simulink model "sim_noise_reduction_R2013a"  (R2013a)
settings: Solver=ode4  SolverMode=SingleTasking  StartTime=0.0  StopTime=10.0  FixedStep=0.001  RelTol=1e-3
libraries: simulink x1
settings Model: CovMetricSettings=dwe  CovHtmlReporting=off  covSaveCumulativeToWorkspaceVar=off  CovSaveSingleToWorkspaceVar=off  CovExternalEMLEnable=on  Creator=kawata  LastModifiedBy=kawata
settings DataIOCC: LimitDataPoints=off  SaveFormat=StructureWithTime
settings DebuggingCC: UnderspecifiedInitializationDetection=Simplified  MergeDetectMultiDrivingBlocksExec=error  SolverPrmCheckMsg=none  FrameProcessingCompatibilityMsg=error  StateNameClashWarn=none  SFUnexpectedBacktrackingDiag=error  SFNoUnconditionalDefaultTransitionDiag=error
settings HardwareCC: ProdBitPerPointer=64  ProdLargestAtomicFloat=Float  ProdIntDivRoundTo=Zero  ProdEndianess=LittleEndian  ProdHWDeviceType=Specified
settings ModelReferenceCC: PropagateSignalLabelsOutOfModel=on
settings GRTTargetCC: CodeReplacementLibrary=C99 (ISO)  GeneratePreprocessorConditionals=Use local settings

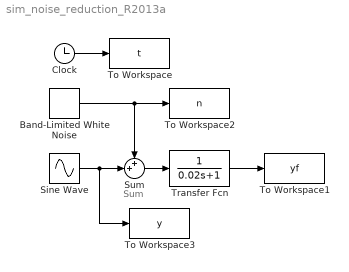
== system sim_noise_reduction_R2013a ==
  note: Sum
  Band-Limited White Noise : simulink/Sources/Band-Limited White Noise  Cov=[1e-5]  Ts=0.001  seed=[23341]
  Clock : Clock
  Sine Wave : Sin  SampleTime=0
  Sum : Sum  Inputs=++|
  To Workspace : ToWorkspace  VariableName=t  SampleTime=-1
  To Workspace1 : ToWorkspace  VariableName=yf  SampleTime=-1
  To Workspace2 : ToWorkspace  VariableName=n  SampleTime=-1
  To Workspace3 : ToWorkspace  VariableName=y  SampleTime=-1
  Transfer Fcn : TransferFcn  Denominator=[0.02 1]
  wires:
  Sine Wave/1 -> To Workspace3/1, Sum/2
  Sum/1 -> Transfer Fcn/1
  Band-Limited White Noise/1 -> To Workspace2/1, Sum/1
  Clock/1 -> To Workspace/1
  Transfer Fcn/1 -> To Workspace1/1
